simulink model "chap02_47"  (R2020a)
settings: Solver=VariableStepAuto  StartTime=0.0  StopTime=10.0  RelTol=1e-3
settings Model: Creator=chen_w3  LastModifiedBy=chen_w3

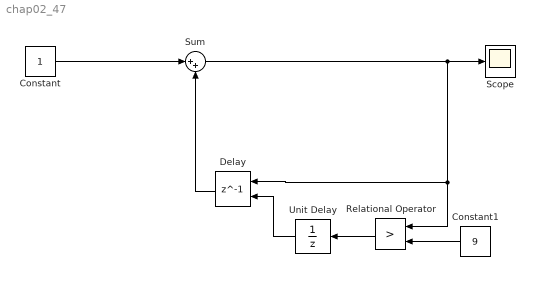
== system chap02_47 ==
  Constant : Constant
  Constant1 : Constant  Value=9
  Delay : Delay  DelayLength=1  InitialCondition=0  ExternalReset=Rising
      settings: InputPortMap=u0,r5
  Relational Operator : RelationalOperator  Operator=>  OutDataTypeStr=boolean  RndMeth=Simplest
  Scope : Scope
  Sum : Sum  Inputs=|++
  Unit Delay : UnitDelay  SampleTime=-1  HasFrameUpgradeWarning=on
  wires:
  Constant/1 -> Sum/1
  Sum/1 -> Delay/1, Relational Operator/1, Scope/1
  Constant1/1 -> Relational Operator/2
  Relational Operator/1 -> Unit Delay/1
  Delay/1 -> Sum/2
  Unit Delay/1 -> Delay/2
